simulink model "ICE"  (R2025b)
settings: Solver=FixedStepAuto  StartTime=0.0  StopTime=10.0  FixedStep=Ts  RelTol=1e-3
values from neighbouring files (symbols this model uses):
  fan_abs_delta = abs(fan_max_factor - fan_min_factor)    [constants.m]
  fan_max_factor = 1    [constants.m]
  fan_min_factor = 0.4    [constants.m]
  ICE_fun_acceleration = 5    [constants.m]
  ICE_fun_deceleration = 5    [constants.m]
  J_ICE = 3.5    [constants.m]
  k_heat = 0.30    (= 0.3)    [constants.m]
  k_radiator = 450.0    (= 450)    [constants.m]
  M_peak = 3500.0    (= 3500)    [constants.m]
  T_amb = 25.0    (= 25)    [constants.m]
  tau = 40.0    (= 40)    [constants.m]
  Ts = 0.001    [constants.m]
settings Model: TunableVars=J_AD,J_ICE,M_AD_nom,P_ballast_nom,P_oil_max,P_oil_min,T_AD_max,T_amb,T_ballast_max,T_cool_max,a_const,ad_fun_acceleration,b_const,k_heat,k_loss,k_loss0,k_rad_AD,k_rad_ballast,k_radiator,omega_ICE_max_prir,omega_ICE_max_run,tau,tau_AD_base,tau_ballast,tau_cool  TunableVarsStorageClass=Auto,Auto,Auto,Auto,Auto,Auto,Auto,Auto,Auto,Auto,Auto,Auto,Auto,Auto,Auto,Auto,Auto,Auto,Auto,Auto,Auto,Auto,Auto,Auto,Auto  TunableVarsTypeQualifier=,,,,,,,,,,,,,,,,,,,,,,,,  Creator=user  LastModifiedBy=user
settings OptimizationCC: DefaultParameterBehavior=Inlined  UseDivisionForNetSlopeComputation=on  GainParamInheritBuiltInType=on  UseFloatMulNetSlope=on  StrengthReduction=on  PassReuseOutputArgsAs=Individual arguments  NoFixptDivByZeroProtection=on  EfficientFloat2IntCast=on  OptimizeBlockOrder=speed  OptimizationPriority=Speed  OptimizationCustomize=off  MultiThreadedLoops=on  AutoScheduleForLoops=on  EfficientTunableParamExpr=on
settings DebuggingCC: ParameterTunabilityLossMsg=error
settings HardwareCC: ProdBitPerLong=64.0  ProdLongLongMode=on  ProdHWDeviceType=Intel->x86-64 (Linux 64)
settings SFSimCC: MATLABDynamicMemAlloc=off  SimTargetLang=C++  SimDLTargetLibrary=mkl-dnn
settings RTWCC: SystemTargetFile=ert.tlc  GenCodeOnly=on  TemplateMakefile=ert_default_tmf  GenerateReport=on  BuildConfiguration=Faster Runs  LaunchReport=on  TargetLang=C++  Description=Embedded Coder
settings CodeAppCC: ForceParamTrailComments=on  IgnoreCustomStorageClasses=off  OperatorAnnotations=on  SimulinkDataObjDesc=on  SFDataObjDesc=on  CustomSymbolStrGlobalVar=rt$N$M  CustomSymbolStrType=$N$M  CustomSymbolStrFcn=$N$M$F  CustomSymbolStrMacro=$N$M  InsertBlockDesc=on
settings ERTTargetCC: InlinedParameterPlacement=Hierarchical  RootIOFormat=Structure reference  ERTCustomFileTemplate=example_file_process.tlc  TargetLangStandard=C++17 (ISO)  GenerateSampleERTMain=on  CodeInterfacePackaging=Reusable function  SupportContinuousTime=on

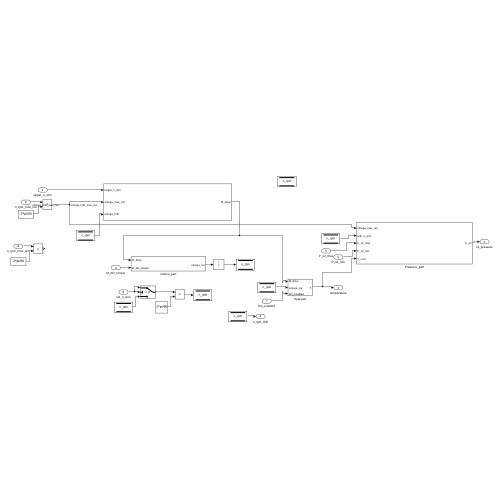
[thumbnail: Simulink's stored preview of the top-level diagram]
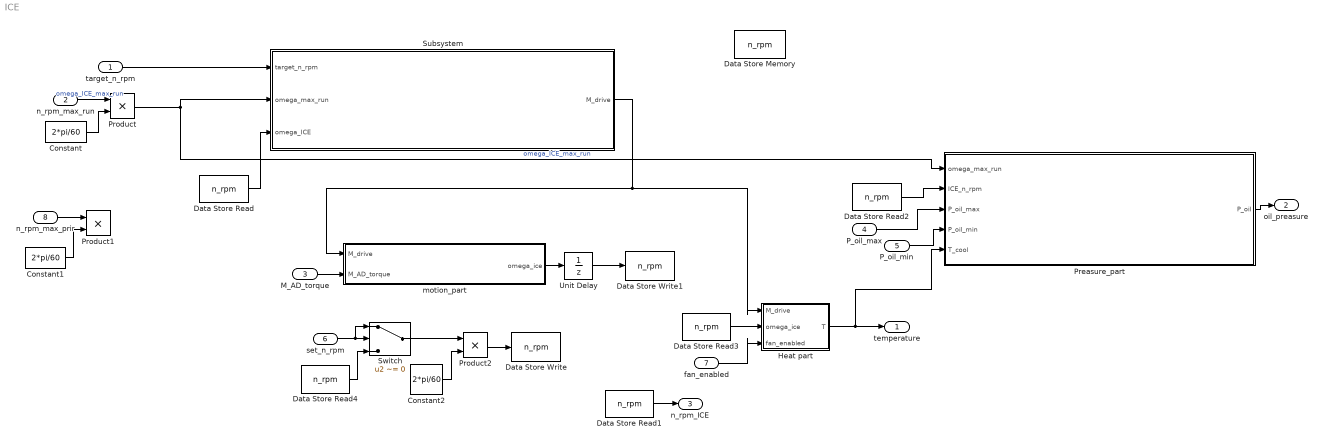
== system ICE ==
  target_n_rpm : Inport
  n_rpm_max_run : Inport  Port=2
  M_AD_torque : Inport  Port=3
  P_oil_max : Inport  Port=4
  P_oil_min : Inport  Port=5
  set_n_rpm : Inport  Port=6
  fan_enabled : Inport  Port=7
  n_rpm_max_prir : Inport  Port=8
  Constant : Constant  Value=2*pi/60
  Constant1 : Constant  Value=2*pi/60
  Constant2 : Constant  Value=2*pi/60
  Data Store Memory : DataStoreMemory  DataStoreName=n_rpm  WriteAfterWriteMsg=warning  ShowAdditionalParam=off
  Data Store Read{,1..4} (5 alike) : DataStoreRead  DataStoreName=n_rpm  IndexOptions=Index vector (dialog)  Indices=1  OutputSizes=1
  Data Store Write : DataStoreWrite  DataStoreName=n_rpm  IndexOptions=Index vector (dialog)  Indices=1  OutputSizes=1
  Data Store Write1 : DataStoreWrite  DataStoreName=n_rpm  IndexOptions=Index vector (dialog)  Indices=1  OutputSizes=1
  Heat part : Subsystem
  Preasure_part : Subsystem
  Product : Product
  Product1 : Product
  Product2 : Product
  Subsystem : Subsystem
  Switch : Switch  Criteria=u2 ~= 0  SaturateOnIntegerOverflow=off  InputSameDT=off
  Unit Delay : UnitDelay  SampleTime=-1  HasFrameUpgradeWarning=on
  motion_part : Subsystem
  temperature : Outport
  oil_preasure : Outport  Port=2
  n_rpm_ICE : Outport  Port=3
  wires:
  target_n_rpm/1 -> Subsystem/1(target_n_rpm)
  Subsystem/1(M_drive) -> Heat part/1(M_drive), motion_part/1(M_drive)
  Product/1 -> Subsystem/2(omega_max_run), Preasure_part/1(omega_max_run)  "omega_ICE_max_run"
  motion_part/1(omega_ice) -> Unit Delay/1
  Heat part/1(T) -> Preasure_part/5(T_cool), temperature/1
  P_oil_max/1 -> Preasure_part/3(P_oil_max)
  Preasure_part/1(P_oil) -> oil_preasure/1
  M_AD_torque/1 -> motion_part/2(M_AD_torque)
  P_oil_min/1 -> Preasure_part/4(P_oil_min)
  Data Store Read/1 -> Subsystem/3(omega_ICE)
  Data Store Read1/1 -> n_rpm_ICE/1
  Data Store Read3/1 -> Heat part/2(omega_ice)
  Unit Delay/1 -> Data Store Write1/1
  Data Store Read2/1 -> Preasure_part/2(ICE_n_rpm)
  fan_enabled/1 -> Heat part/3(fan_enabled)
  set_n_rpm/1 -> Switch/1, Switch/2
  Data Store Read4/1 -> Switch/3
  Constant/1 -> Product/2
  n_rpm_max_run/1 -> Product/1  "omega_ICE_max_run"
  n_rpm_max_prir/1 -> Product1/1
  Constant1/1 -> Product1/2
  Switch/1 -> Product2/1
  Constant2/1 -> Product2/2
  Product2/1 -> Data Store Write/1

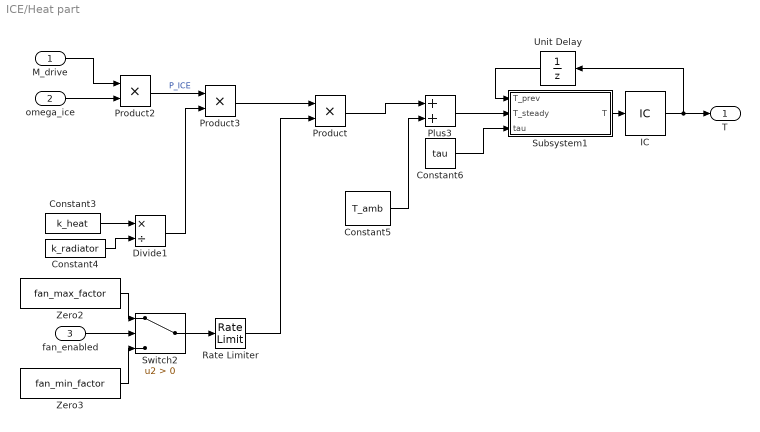
== system ICE/Heat part ==
  M_drive : Inport
  omega_ice : Inport  Port=2
  fan_enabled : Inport  Port=3
  Constant3 : Constant  Value=k_heat
  Constant4 : Constant  Value=k_radiator
  Constant5 : Constant  Value=T_amb
  Constant6 : Constant  Value=tau
  Divide1 : Product  Inputs=*/
  IC : InitialCondition  Value=T_amb
  Plus3 : Sum
  Product : Product
  Product2 : Product
  Product3 : Product
  Rate Limiter : RateLimiter  RisingSlewLimit=fan_abs_delta/ICE_fun_acceleration  FallingSlewLimit=-fan_abs_delta/ICE_fun_deceleration
  Subsystem1 : Subsystem
  Switch2 : Switch  Criteria=u2 > Threshold  SaturateOnIntegerOverflow=off  InputSameDT=off
  Unit Delay : UnitDelay  InitialCondition=T_amb  SampleTime=-1  HasFrameUpgradeWarning=on
  Zero2 : Constant  Value=fan_max_factor  OutDataTypeStr=Inherit: Inherit via back propagation
  Zero3 : Constant  Value=fan_min_factor  OutDataTypeStr=Inherit: Inherit via back propagation
  T : Outport
  wires:
  omega_ice/1 -> Product2/2
  Constant3/1 -> Divide1/1
  Constant4/1 -> Divide1/2
  Divide1/1 -> Product3/2
  Constant5/1 -> Plus3/2
  Product2/1 -> Product3/1  "P_ICE"
  Plus3/1 -> Subsystem1/2(T_steady)
  M_drive/1 -> Product2/1
  Unit Delay/1 -> Subsystem1/1(T_prev)
  Subsystem1/1(T) -> IC/1
  IC/1 -> Unit Delay/1, T/1
  Zero3/1 -> Switch2/3
  Zero2/1 -> Switch2/1
  fan_enabled/1 -> Switch2/2
  Product3/1 -> Product/1
  Product/1 -> Plus3/1
  Switch2/1 -> Rate Limiter/1
  Constant6/1 -> Subsystem1/3(tau)
  Rate Limiter/1 -> Product/2

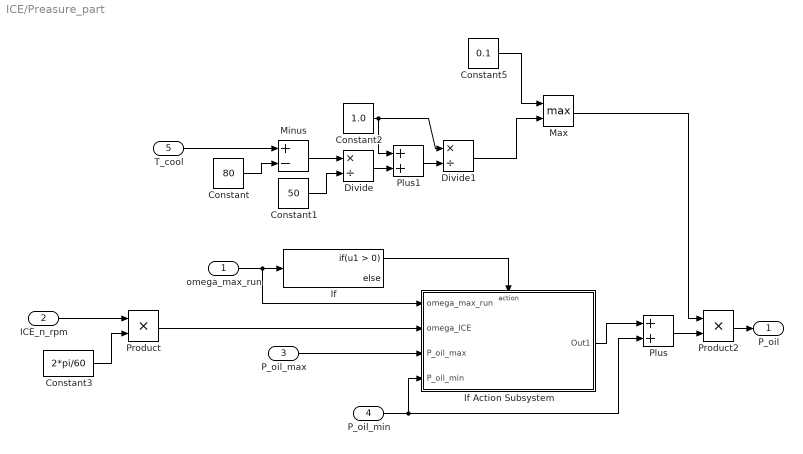
== system ICE/Preasure_part ==
  omega_max_run : Inport
  ICE_n_rpm : Inport  Port=2
  P_oil_max : Inport  Port=3
  P_oil_min : Inport  Port=4
  T_cool : Inport  Port=5
  Constant : Constant  Value=80
  Constant1 : Constant  Value=50
  Constant2 : Constant  Value=1.0
  Constant3 : Constant  Value=2*pi/60
  Constant5 : Constant  Value=0.1  OutDataTypeStr=Inherit: Inherit via back propagation
  Divide : Product  Inputs=*/
  Divide1 : Product  Inputs=*/
  If : If
  If Action Subsystem : Subsystem  TreatAsAtomicUnit=on
  Max : MinMax  Function=max  Inputs=2
  Minus : Sum  Inputs=+-
  Plus : Sum
  Plus1 : Sum
  Product : Product
  Product2 : Product
  P_oil : Outport
  wires:
  Product2/1 -> P_oil/1
  Constant5/1 -> Max/1
  P_oil_min/1 -> If Action Subsystem/4(P_oil_min), Plus/2
  Max/1 -> Product2/1
  If Action Subsystem/1(Out1) -> Plus/1
  Divide1/1 -> Max/2
  Plus/1 -> Product2/2
  omega_max_run/1 -> If Action Subsystem/1(omega_max_run), If/1
  If/1 -> If Action Subsystem/Action
  P_oil_max/1 -> If Action Subsystem/3(P_oil_max)
  Constant/1 -> Minus/2
  T_cool/1 -> Minus/1
  Minus/1 -> Divide/1
  Constant1/1 -> Divide/2
  Divide/1 -> Plus1/2
  Plus1/1 -> Divide1/2
  Constant2/1 -> Divide1/1, Plus1/1
  Constant3/1 -> Product/2
  ICE_n_rpm/1 -> Product/1
  Product/1 -> If Action Subsystem/2(omega_ICE)

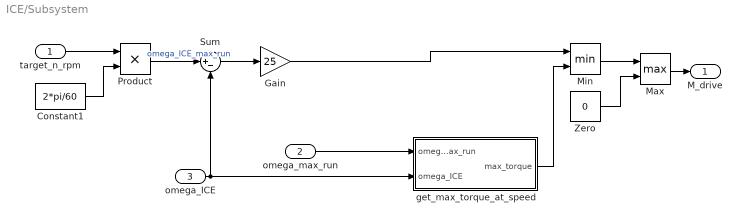
== system ICE/Subsystem ==
  target_n_rpm : Inport
  omega_max_run : Inport  Port=2
  omega_ICE : Inport  Port=3
  Constant1 : Constant  Value=2*pi/60
  Gain : Gain  Gain=25
  Max : MinMax  Function=max  Inputs=2
  Min : MinMax  Inputs=2
  Product : Product
  Sum : Sum  Inputs=|+-
  Zero : Constant  Value=0  OutDataTypeStr=Inherit: Inherit via back propagation
  get_max_torque_at_speed : Subsystem
  M_drive : Outport
  wires:
  get_max_torque_at_speed/1(max_torque) -> Min/2
  Zero/1 -> Max/2
  Min/1 -> Max/1
  Max/1 -> M_drive/1
  omega_max_run/1 -> get_max_torque_at_speed/1(omega_ICE_max_run)
  omega_ICE/1 -> get_max_torque_at_speed/2(omega_ICE), Sum/2
  Sum/1 -> Gain/1
  Gain/1 -> Min/1
  target_n_rpm/1 -> Product/1
  Constant1/1 -> Product/2
  Product/1 -> Sum/1  "omega_ICE_max_run"

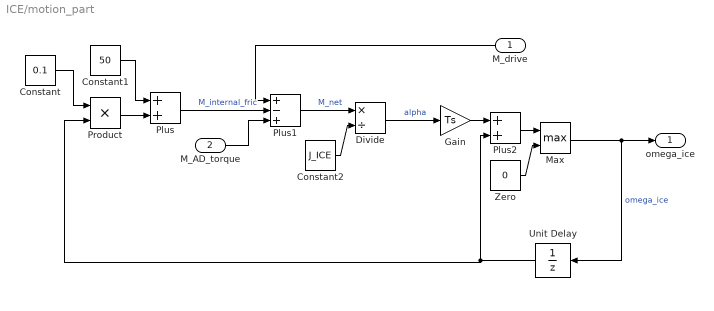
== system ICE/motion_part ==
  M_drive : Inport
  M_AD_torque : Inport  Port=2
  Constant : Constant  Value=0.1
  Constant1 : Constant  Value=50
  Constant2 : Constant  Value=J_ICE
  Divide : Product  Inputs=*/
  Gain : Gain  Gain=Ts
  Max : MinMax  Function=max  Inputs=2
  Plus : Sum
  Plus1 : Sum  Inputs=+-+
  Plus2 : Sum
  Product : Product
  Unit Delay : UnitDelay  SampleTime=-1  HasFrameUpgradeWarning=on
  Zero : Constant  Value=0  OutDataTypeStr=Inherit: Inherit via back propagation
  omega_ice : Outport
  wires:
  M_drive/1 -> Plus1/1
  Max/1 -> Unit Delay/1, omega_ice/1  "omega_ice"
  Constant1/1 -> Plus/1
  Divide/1 -> Gain/1  "alpha"
  M_AD_torque/1 -> Plus1/3
  Gain/1 -> Plus2/1
  Product/1 -> Plus/2
  Zero/1 -> Max/2
  Constant2/1 -> Divide/2
  Plus1/1 -> Divide/1  "M_net"
  Plus2/1 -> Max/1
  Constant/1 -> Product/1
  Plus/1 -> Plus1/2  "M_internal_fric"
  Unit Delay/1 -> Product/2, Plus2/2

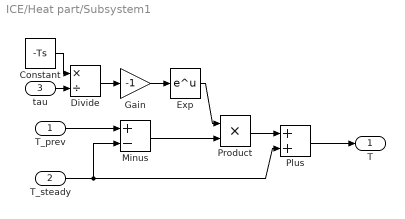
== system ICE/Heat part/Subsystem1 ==
  T_prev : Inport
  T_steady : Inport  Port=2
  tau : Inport  Port=3
  Constant : Constant  Value=-Ts
  Divide : Product  Inputs=*/
  Exp : Math
  Gain : Gain  Gain=-1
  Minus : Sum  Inputs=+-
  Plus : Sum
  Product : Product
  T : Outport
  wires:
  T_prev/1 -> Minus/1
  T_steady/1 -> Plus/2, Minus/2
  Minus/1 -> Product/2
  Exp/1 -> Product/1
  Product/1 -> Plus/1
  Plus/1 -> T/1
  Divide/1 -> Gain/1
  Gain/1 -> Exp/1
  Constant/1 -> Divide/1
  tau/1 -> Divide/2

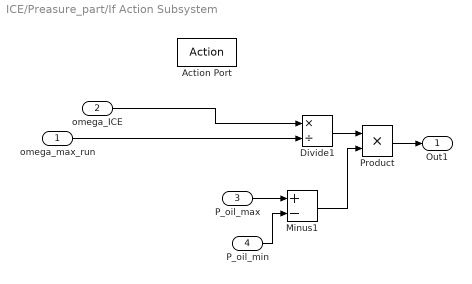
== system ICE/Preasure_part/If Action Subsystem ==
  omega_max_run : Inport
  omega_ICE : Inport  Port=2
  P_oil_max : Inport  Port=3
  P_oil_min : Inport  Port=4
  Action Port : ActionPort  ActionPortLabel=if(u1 > 0)
  Divide1 : Product  Inputs=*/
  Minus1 : Sum  Inputs=+-
  Product : Product
  Out1 : Outport
  wires:
  Minus1/1 -> Product/2
  P_oil_max/1 -> Minus1/1
  omega_ICE/1 -> Divide1/1
  omega_max_run/1 -> Divide1/2
  P_oil_min/1 -> Minus1/2
  Divide1/1 -> Product/1
  Product/1 -> Out1/1

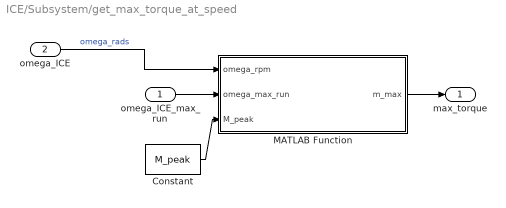
== system ICE/Subsystem/get_max_torque_at_speed ==
  omega_ICE_max_run : Inport
  omega_ICE : Inport  Port=2
  Constant : Constant  Value=M_peak
  MATLAB Function : MATLAB Function  TreatAsAtomicUnit=on
  max_torque : Outport
  wires:
  omega_ICE_max_run/1 -> MATLAB Function/2(omega_max_run)
  MATLAB Function/1(m_max) -> max_torque/1
  Constant/1 -> MATLAB Function/3(M_peak)
  omega_ICE/1 -> MATLAB Function/1(omega_rpm)  "omega_rads"

== matlab function ICE/Subsystem/get_max_torque_at_speed/MATLAB Function ==
  data: omega_rpm input; omega_max_run input; m_max output; M_peak input
function m_max = torque_limit(omega_rpm, omega_max_run, M_peak)

thresh1 = omega_max_run * 0.45;
thresh2 = omega_max_run * 0.8;
thresh3 = omega_max_run;

if omega_rpm < thresh1
    m_max = M_peak / 7 * (1 + 6 * (omega_rpm / thresh1));
elseif omega_rpm < thresh2
    m_max = M_peak;
elseif omega_rpm < thresh3
    ratio = (omega_rpm - thresh2) / (thresh3 - thresh2);
    m_max = M_peak * (1.0 - ratio * 0.25);
else
    m_max = M_peak * 0.75;
end
end
